simulink model "sampleModel106"  (R2022a)
settings: Solver=VariableStepAuto  StartTime=0.0  StopTime=10.0  RelTol=1e-3
undefined symbols (not defined in the file): DiscIntNeverNeededParam, magnitude, Newton, Raphson
libraries: simulink x379, slpidlib x89
(part 6 of 16)

== system sampleModel106/cfblk86/cfblk12/cfblk6 ==
  cfblk1 : Inport
  cfblk10 : Inport  Port=2
  cfblk11 : Inport  Port=3
  cfblk{14..17} (4 alike) : Delay
  cfblk3 : Delay  ShowEnablePort=on
      settings: InputPortMap=u0,e6
  cfblk4 : slpidlib/PID Controller (2DOF)  Controller=PID  Form=Parallel  TimeDomain=Discrete-time  UseExternalTs=off  SampleTime=-1  IntegratorMethod=Forward Euler  FilterMethod=Forward Euler  ControllerParametersSource=internal  P=1  I=1  UseKiTs=off  D=0  N=100  UseFilter=on  b=1  c=1  TunerSelectOption=Transfer Function Based (PID Tuner App)  InitialConditionSource=internal  InitialConditionForIntegrator=0  InitialConditionForFilter=0  DifferentiatorICPrevScaledInput=0  ExternalReset=none  TrackingMode=off  Kt=1  LimitOutput=off  SatLimitsSource=internal  UpperSaturationLimit=inf  LowerSaturationLimit=-inf  LinearizeAsGain=off  AntiWindupMode=none  Kb=1  POutMin=[]  POutMax=[]  IOutMin=[]  IOutMax=[]  DOutMin=[]  DOutMax=[]  NOutMin=[]  NOutMax=[]  bOutMin=[]  bOutMax=[]  cOutMin=[]  cOutMax=[]  SumOutMin=[]  SumOutMax=[]  SaturationOutMin=[]  SaturationOutMax=[]  PParamMin=[]  PParamMax=[]  IParamMin=[]  IParamMax=[]  DParamMin=[]  DParamMax=[]  NParamMin=[]  NParamMax=[]  bParamMin=[]  bParamMax=[]  cParamMin=[]  cParamMax=[]  KbParamMin=[]  KbParamMax=[]  KtParamMin=[]  KtParamMax=[]  KbOutMin=[]  KbOutMax=[]  KtOutMin=[]  KtOutMax=[]  IntegratorOutMin=[]  IntegratorOutMax=[]  FilterOutMin=[]  FilterOutMax=[]  SumI1OutMin=[]  SumI1OutMax=[]  SumI2OutMin=[]  SumI2OutMax=[]  SumI3OutMin=[]  SumI3OutMax=[]  SumI4OutMin=[]  SumI4OutMax=[]  SumDOutMin=[]  SumDOutMax=[]  Sum1OutMin=[]  Sum1OutMax=[]  Sum2OutMin=[]  Sum2OutMax=[]  Sum3OutMin=[]  Sum3OutMax=[]  DifferentiatorOutMin=[]  DifferentiatorOutMax=[]  FilterDiffOutCoefMin=[]  FilterDiffOutCoefMax=[]  ReciprocalOutMin=[]  ReciprocalOutMax=[]  SumDenOutMin=[]  SumDenOutMax=[]  SumNumOutMin=[]  SumNumOutMax=[]  DivideOutMin=[]  DivideOutMax=[]  UdiffTsProdOutMin=[]  UdiffTsProdOutMax=[]  NTsProdOutMin=[]  NTsProdOutMax=[]  UintegralTsProdOutMin=[]  UintegralTsProdOutMax=[]  UngainTsProdOutMin=[]  UngainTsProdOutMax=[]  IntegratorContinuousStateAttributes=''  IntegratorStateMustResolveToSignalObject=off  IntegratorRTWStateStorageClass=Auto  FilterContinuousStateAttributes=''  FilterStateMustResolveToSignalObject=off  FilterRTWStateStorageClass=Auto  ParallelPVariant=InternalParameters  IdealPVariant=Disabled  IVariant=InternalParameters  DVariant=InternalParameters  bVariant=InternalParameters  cVariant=InternalParameters  IntegratorVariant=Discrete  SatVariant=Disabled  AWVariant=Passthrough  PCopyVariant=Disabled  TRVariant=Disabled  FdbkBlocksVariant=Forward  IdealPFdbkVariant=Disabled  SatFdbkVariant=Disabled  DerivativeFilterVariant=ForwardEulerFilter  NVariant=InternalParameters  NCopyVariant=Disabled  FilterICVariant=InternalICsFilter  IntegratorICVariant=InternalICs  ExternalResetVariant=Disabled  TRSumVariant=Passthrough  SumFdbkVariant=Disabled  SumVariant=Sum_PID  TsampFilterVariant=InternalTs  TsampNgainVariant=Passthrough  TsampIntegralVariant=Passthrough  ExternalSaturationOutDataTypeStr=Inherit: Same as second input
      settings: SourceProductBaseCode=SL
  cfblk5 : Signum
  cfblk6 : Subsystem
  cfblk7 : Subsystem
  cfblk8 : Subsystem
  cfblk9 : Subsystem
  cfblk2 : Outport
  cfblk12 : Outport  Port=2
  cfblk13 : Outport  Port=3
  wires:
  cfblk10/1 -> cfblk9/1(cfblk1)
  cfblk7/1(cfblk2) -> cfblk9/2(cfblk7)
  cfblk7/2(cfblk9) -> cfblk8/1(cfblk1)
  cfblk4/1 -> cfblk3/1, cfblk7/3(cfblk8)
  cfblk8/2(cfblk8) -> cfblk2/1
  cfblk11/1 -> cfblk12/1
  cfblk3/1 -> cfblk5/1
  cfblk1/1 -> cfblk4/1
  cfblk5/1 -> cfblk9/3(cfblk8)
  cfblk7/3(cfblk10) -> cfblk9/4(cfblk9)
  cfblk9/2(cfblk10) -> cfblk6/1(cfblk1)
  cfblk6/1(cfblk2) -> cfblk13/1
  cfblk9/1(cfblk2) -> cfblk14/1
  cfblk14/1 -> cfblk3/2
  cfblk8/1(cfblk2) -> cfblk15/1
  cfblk15/1 -> cfblk7/1(cfblk1)
  cfblk8/3(cfblk9) -> cfblk16/1
  cfblk16/1 -> cfblk7/2(cfblk7)
  cfblk7/4(cfblk11) -> cfblk17/1
  cfblk17/1 -> cfblk4/2

== system sampleModel106/cfblk86/cfblk12/cfblk7 ==
  cfblk1 : Inport
  cfblk9 : Inport  Port=2
  cfblk10 : Inport  Port=3
  cfblk11 : Inport  Port=4
  cfblk12 : Inport  Port=5
  cfblk13 : Inport  Port=6
  cfblk15 : Delay
  cfblk16 : Delay
  cfblk17 : Delay
  cfblk3 : Abs  SaturateOnIntegerOverflow=off
  cfblk4 : Sum  Inputs=-+
  cfblk5 : DotProduct  OutDataTypeStr=Inherit: Inherit via internal rule
  cfblk6 : ComplexToMagnitudeAngle
  cfblk7 : Subsystem
  cfblk8 : Subsystem
  cfblk2 : Outport
  cfblk14 : Outport  Port=2
  wires:
  cfblk1/1 -> cfblk5/1
  cfblk7/1(cfblk2) -> cfblk3/1
  cfblk12/1 -> cfblk4/1
  cfblk13/1 -> cfblk4/2
  cfblk9/1 -> cfblk14/1
  cfblk11/1 -> cfblk6/1
  cfblk4/1 -> cfblk7/2(cfblk12)
  cfblk10/1 -> cfblk2/1
  cfblk5/1 -> cfblk8/2(cfblk11)
  cfblk6/1 -> cfblk7/3(cfblk13)
  cfblk8/1(cfblk2) -> cfblk7/4(cfblk14)
  cfblk3/1 -> cfblk15/1
  cfblk15/1 -> cfblk7/1(cfblk1)
  cfblk7/2(cfblk15) -> cfblk16/1
  cfblk16/1 -> cfblk5/2
  cfblk7/3(cfblk16) -> cfblk17/1
  cfblk17/1 -> cfblk8/1(cfblk1)

== system sampleModel106/cfblk86/cfblk12/cfblk8 ==
  cfblk1 : Inport
  cfblk11 : Inport  Port=2
  cfblk12 : Inport  Port=3
  cfblk10 : Subsystem
  cfblk13 : Delay
  cfblk3 : Delay
  cfblk4 : simulink/Discrete/Transfer Fcn First Order  PoleZ=0.95  ICPrevOutput=0.0  DoSatur=off
  cfblk5 : DiscreteFilter
  cfblk6 : ComplexToMagnitudeAngle
  cfblk7 : Abs  SaturateOnIntegerOverflow=off
  cfblk8 : Sqrt
  cfblk9 : Constant  Value=[-768190437.472852]  SampleTime=1
  cfblk2 : Outport
  wires:
  cfblk1/1 -> cfblk10/2(cfblk7)
  cfblk4/1 -> cfblk3/1
  cfblk11/1 -> cfblk6/1
  cfblk10/1(cfblk2) -> cfblk4/1
  cfblk10/2(cfblk11) -> cfblk2/1
  cfblk12/1 -> cfblk10/3(cfblk8)
  cfblk5/1 -> cfblk10/4(cfblk9)
  cfblk10/3(cfblk12) -> cfblk8/1
  cfblk9/1 -> cfblk7/1
  cfblk6/1 -> cfblk5/1
  cfblk7/1 -> cfblk10/5(cfblk10)
  cfblk3/1 -> cfblk13/1
  cfblk13/1 -> cfblk10/1(cfblk1)

== system sampleModel106/cfblk86/cfblk12/cfblk9 ==
  cfblk1 : Inport
  cfblk8 : Inport  Port=2
  cfblk10 : Delay
  cfblk11 : Delay
  cfblk3 : simulink/Discrete/Difference  ICPrevInput=0.0  OutMin=[]  OutMax=[]  OutDataTypeStr=Inherit: Inherit via back propagation  OutDataType=fixdt(1, 16)  OutScaling=2^-10  DoSatur=off
  cfblk4 : simulink/Math Operations/MinMax Running Resettable  Function=min  vinit=0.0
  cfblk5 : Gain  Gain=[726512921.677245]
  cfblk6 : ComplexToMagnitudeAngle
  cfblk7 : Subsystem
  cfblk9 : Delay
  cfblk2 : Outport
  wires:
  cfblk8/1 -> cfblk7/1(cfblk1)
  cfblk3/1 -> cfblk4/1
  cfblk5/1 -> cfblk7/3(cfblk15)
  cfblk7/1(cfblk2) -> cfblk4/2
  cfblk7/2(cfblk16) -> cfblk6/1
  cfblk1/1 -> cfblk2/1
  cfblk4/1 -> cfblk9/1
  cfblk9/1 -> cfblk3/1
  cfblk6/1 -> cfblk10/1
  cfblk10/1 -> cfblk5/1
  cfblk6/2 -> cfblk11/1
  cfblk11/1 -> cfblk7/2(cfblk14)

== system sampleModel106/cfblk86/cfblk13/cfblk5 ==
  cfblk1 : Inport
  cfblk13 : Inport  Port=2
  cfblk10 : Sin  TimeSource=Use external signal  SampleTime=0
  cfblk11 : Subsystem
  cfblk12 : Subsystem
  cfblk15 : Delay
  cfblk16 : Delay
  cfblk3 : Delay  ShowEnablePort=on
      settings: InputPortMap=u0,e6
  cfblk4 : DiscreteIntegrator  SampleTime=-1  ICPrevOutput=DiscIntNeverNeededParam  ICPrevScaledInput=DiscIntNeverNeededParam
  cfblk5 : Sum  Inputs=+-
  cfblk6 : Trigonometry
  cfblk7 : Trigonometry
  cfblk8 : Sum  Inputs=|++
  cfblk9 : Reshape
  cfblk2 : Outport
  cfblk14 : Outport  Port=2
  wires:
  cfblk13/1 -> cfblk8/1, cfblk11/3(cfblk10)
  cfblk8/1 -> cfblk7/1
  cfblk11/1(cfblk2) -> cfblk12/1(cfblk1)
  cfblk10/1 -> cfblk5/1
  cfblk7/1 -> cfblk6/1, cfblk5/2
  cfblk5/1 -> cfblk9/1
  cfblk9/1 -> cfblk2/1, cfblk15/1
  cfblk3/1 -> cfblk11/1(cfblk1), cfblk11/2(cfblk9)
  cfblk4/1 -> cfblk12/2(cfblk8), cfblk14/1
  cfblk12/1(cfblk2) -> cfblk10/1
  cfblk12/2(cfblk10) -> cfblk8/2
  cfblk1/1 -> cfblk3/2, cfblk4/1
  cfblk15/1 -> cfblk12/3(cfblk9)
  cfblk6/1 -> cfblk16/1
  cfblk16/1 -> cfblk3/1

== system sampleModel106/cfblk86/cfblk13/cfblk6 ==
  cfblk1 : Inport
  cfblk7 : Inport  Port=2
  cfblk8 : Inport  Port=3
  cfblk9 : Inport  Port=4
  cfblk3 : Sum  Inputs=+
  cfblk4 : Sum  Inputs=+
  cfblk5 : Constant  Value=[176043133.262875]  SampleTime=1
  cfblk6 : Subsystem
  cfblk2 : Outport
  wires:
  cfblk9/1 -> cfblk2/1
  cfblk8/1 -> cfblk3/1
  cfblk4/1 -> cfblk6/1(cfblk1)
  cfblk3/1 -> cfblk4/1
  cfblk5/1 -> cfblk6/2(cfblk5)

== system sampleModel106/cfblk86/cfblk13/cfblk7 ==
  cfblk1 : Inport
  cfblk7 : Inport  Port=2
  cfblk8 : Inport  Port=3
  cfblk10 : Delay
  cfblk3 : Constant  Value=[-929390483.160695]  SampleTime=1
  cfblk4 : Subsystem
  cfblk5 : Subsystem
  cfblk6 : Subsystem
  cfblk9 : Delay
  cfblk2 : Outport
  wires:
  cfblk8/1 -> cfblk4/1(cfblk1)
  cfblk5/1(cfblk2) -> cfblk4/2(cfblk11)
  cfblk1/1 -> cfblk2/1
  cfblk3/1 -> cfblk5/1(cfblk1)
  cfblk5/2(cfblk12) -> cfblk6/1(cfblk1)
  cfblk7/1 -> cfblk6/2(cfblk13)
  cfblk4/1(cfblk2) -> cfblk9/1
  cfblk9/1 -> cfblk5/3(cfblk11)
  cfblk6/1(cfblk2) -> cfblk10/1
  cfblk10/1 -> cfblk5/2(cfblk10)

== system sampleModel106/cfblk86/cfblk9/cfblk8 ==
  cfblk1 : Inport
  cfblk10 : Subsystem
  cfblk11 : Subsystem
  cfblk{3,12..15} (5 alike) : Delay
  cfblk4 : DiscreteStateSpace  SampleTime=-1
  cfblk5 : Product
  cfblk6 : Math  Operator=log10
  cfblk7 : ComplexToMagnitudeAngle
  cfblk8 : Subsystem
  cfblk9 : Subsystem
  cfblk2 : Outport
  wires:
  cfblk10/1(cfblk2) -> cfblk9/2(cfblk13)
  cfblk3/1 -> cfblk4/1, cfblk2/1
  cfblk6/1 -> cfblk3/1
  cfblk7/1 -> cfblk8/1(cfblk1)
  cfblk8/1(cfblk2) -> cfblk9/3(cfblk14)
  cfblk9/1(cfblk2) -> cfblk11/1(cfblk1)
  cfblk1/1 -> cfblk6/1, cfblk8/3(cfblk7), cfblk8/4(cfblk8), cfblk10/4(cfblk11)
  cfblk9/2(cfblk15) -> cfblk11/2(cfblk11)
  cfblk8/2(cfblk12) -> cfblk5/1
  cfblk7/2 -> cfblk10/1(cfblk1), cfblk10/3(cfblk10), cfblk8/7(cfblk11)
  cfblk10/3(cfblk14) -> cfblk14/1, cfblk15/1
  cfblk4/1 -> cfblk7/1, cfblk8/6(cfblk10)
  cfblk5/1 -> cfblk10/2(cfblk9), cfblk10/5(cfblk12)
  cfblk11/1(cfblk2) -> cfblk12/1
  cfblk12/1 -> cfblk9/1(cfblk1)
  cfblk10/2(cfblk13) -> cfblk13/1
  cfblk13/1 -> cfblk8/2(cfblk6)
  cfblk14/1 -> cfblk5/2
  cfblk15/1 -> cfblk8/5(cfblk9)

== system sampleModel106/cfblk87/cfblk7/cfblk10 ==
  cfblk1 : Inport
  cfblk6 : Inport  Port=2
  cfblk3 : Assignment  DiagnosticForDimensions=Warning  IndexOptions=Index vector (dialog)  Indices=1  OutputSizes=1
  cfblk4 : Constant  Value=[-447952016.572261]  SampleTime=1
  cfblk5 : Subsystem
  cfblk8 : Delay
  cfblk2 : Outport
  cfblk7 : Outport  Port=2
  wires:
  cfblk6/1 -> cfblk7/1
  cfblk4/1 -> cfblk2/1, cfblk5/3(cfblk15)
  cfblk5/1(cfblk2) -> cfblk3/1
  cfblk1/1 -> cfblk5/2(cfblk14)
  cfblk5/2(cfblk16) -> cfblk3/2
  cfblk3/1 -> cfblk8/1
  cfblk8/1 -> cfblk5/1(cfblk1)

== system sampleModel106/cfblk87/cfblk7/cfblk11 ==
  cfblk1 : Inport
  cfblk7 : Inport  Port=2
  cfblk3 : Product  Inputs=**
  cfblk4 : Reshape
  cfblk5 : Constant  Value=[-816487384.048334]  SampleTime=1
  cfblk6 : Subsystem
  cfblk2 : Outport
  cfblk8 : Outport  Port=2
  wires:
  cfblk5/1 -> cfblk4/1
  cfblk6/1(cfblk2) -> cfblk3/1
  cfblk1/1 -> cfblk2/1
  cfblk4/1 -> cfblk3/2
  cfblk7/1 -> cfblk6/1(cfblk1)
  cfblk3/1 -> cfblk8/1

== system sampleModel106/cfblk87/cfblk8/cfblk10 ==
  cfblk1 : Inport
  cfblk10 : Subsystem  TreatAsAtomicUnit=on
  cfblk11 : Subsystem  TreatAsAtomicUnit=on
  cfblk{12..18} (7 alike) : Delay
  cfblk3 : simulink/Discrete/Tapped Delay  vinit=0.0  samptime=-1  NumDelays=1  DelayOrder=Oldest  includeCurrent=off
  cfblk4 : Subsystem
  cfblk5 : Subsystem
  cfblk6 : If  IfExpression=u1 >= 0  SampleTime=1
  cfblk7 : If  IfExpression=u1 >= 0  SampleTime=1
  cfblk8 : Subsystem  TreatAsAtomicUnit=on
  cfblk9 : Subsystem  TreatAsAtomicUnit=on
  cfblk2 : Outport
  wires:
  cfblk11/1(cfblk2) -> cfblk4/1(cfblk1)
  cfblk10/1(cfblk2) -> cfblk5/1(cfblk1), cfblk18/1
  cfblk1/1 -> cfblk6/1, cfblk11/2(cfblk10), cfblk2/1
  cfblk9/1(cfblk2) -> cfblk3/1
  cfblk5/2(cfblk15) -> cfblk16/1, cfblk17/1
  cfblk8/1(cfblk2) -> cfblk11/1(cfblk1)
  cfblk6/1 -> cfblk8/Action
  cfblk6/2 -> cfblk9/Action
  cfblk7/1 -> cfblk10/Action
  cfblk7/2 -> cfblk11/Action
  cfblk4/1(cfblk2) -> cfblk12/1
  cfblk12/1 -> cfblk10/1(cfblk1)
  cfblk5/1(cfblk2) -> cfblk13/1
  cfblk13/1 -> cfblk9/2(cfblk14)
  cfblk3/1 -> cfblk14/1
  cfblk14/1 -> cfblk9/1(cfblk1)
  cfblk9/2(cfblk15) -> cfblk15/1
  cfblk15/1 -> cfblk7/1
  cfblk16/1 -> cfblk8/1(cfblk1)
  cfblk17/1 -> cfblk11/3(cfblk11)
  cfblk18/1 -> cfblk8/2(cfblk9)

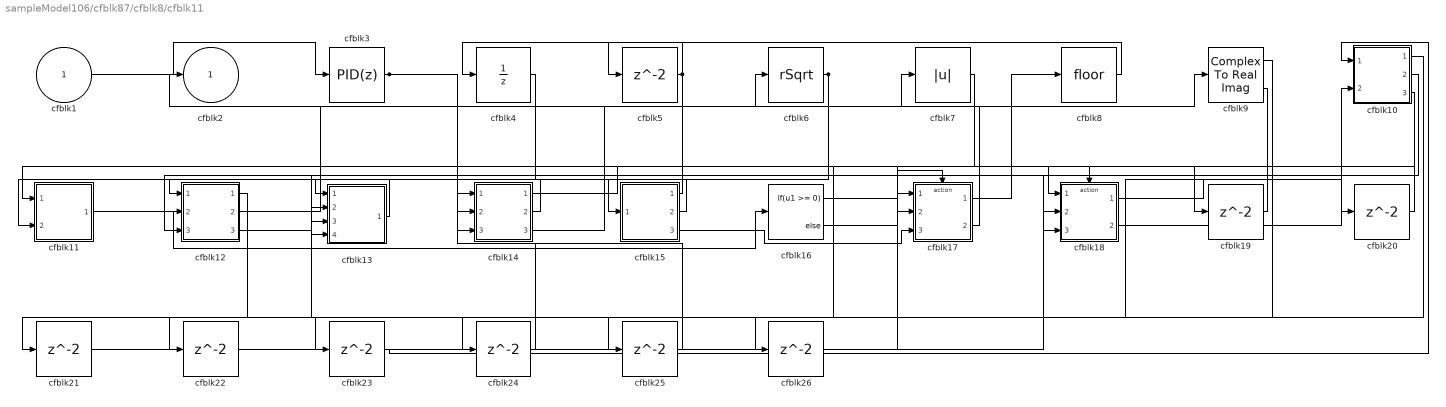
== system sampleModel106/cfblk87/cfblk8/cfblk11 ==
  cfblk1 : Inport
  cfblk10 : Subsystem
  cfblk11 : Subsystem
  cfblk12 : Subsystem
  cfblk13 : Subsystem
  cfblk14 : Subsystem
  cfblk15 : Subsystem
  cfblk16 : If  IfExpression=u1 >= 0  SampleTime=1
  cfblk17 : Subsystem  TreatAsAtomicUnit=on
  cfblk18 : Subsystem  TreatAsAtomicUnit=on
  cfblk{5,19..26} (9 alike) : Delay
  cfblk3 : slpidlib/PID Controller  Controller=PID  Form=Parallel  TimeDomain=Discrete-time  UseExternalTs=off  SampleTime=-1  IntegratorMethod=Forward Euler  FilterMethod=Forward Euler  ControllerParametersSource=internal  P=1  I=1  UseKiTs=off  D=0  N=100  UseFilter=on  TunerSelectOption=Transfer Function Based (PID Tuner App)  InitialConditionSource=internal  InitialConditionForIntegrator=0  InitialConditionForFilter=0  DifferentiatorICPrevScaledInput=0  ExternalReset=none  TrackingMode=off  Kt=1  LimitOutput=off  SatLimitsSource=internal  UpperSaturationLimit=inf  LowerSaturationLimit=-inf  LinearizeAsGain=off  AntiWindupMode=none  Kb=1  POutMin=[]  POutMax=[]  IOutMin=[]  IOutMax=[]  DOutMin=[]  DOutMax=[]  NOutMin=[]  NOutMax=[]  SumOutMin=[]  SumOutMax=[]  SaturationOutMin=[]  SaturationOutMax=[]  PParamMin=[]  PParamMax=[]  IParamMin=[]  IParamMax=[]  DParamMin=[]  DParamMax=[]  NParamMin=[]  NParamMax=[]  KbParamMin=[]  KbParamMax=[]  KtParamMin=[]  KtParamMax=[]  KbOutMin=[]  KbOutMax=[]  KtOutMin=[]  KtOutMax=[]  IntegratorOutMin=[]  IntegratorOutMax=[]  FilterOutMin=[]  FilterOutMax=[]  SumI1OutMin=[]  SumI1OutMax=[]  SumI2OutMin=[]  SumI2OutMax=[]  SumI3OutMin=[]  SumI3OutMax=[]  SumI4OutMin=[]  SumI4OutMax=[]  SumDOutMin=[]  SumDOutMax=[]  DifferentiatorOutMin=[]  DifferentiatorOutMax=[]  FilterDiffOutCoefMin=[]  FilterDiffOutCoefMax=[]  ReciprocalOutMin=[]  ReciprocalOutMax=[]  SumDenOutMin=[]  SumDenOutMax=[]  SumNumOutMin=[]  SumNumOutMax=[]  DivideOutMin=[]  DivideOutMax=[]  UdiffTsProdOutMin=[]  UdiffTsProdOutMax=[]  NTsProdOutMin=[]  NTsProdOutMax=[]  UintegralTsProdOutMin=[]  UintegralTsProdOutMax=[]  UngainTsProdOutMin=[]  UngainTsProdOutMax=[]  IntegratorContinuousStateAttributes=''  IntegratorStateMustResolveToSignalObject=off  IntegratorRTWStateStorageClass=Auto  FilterContinuousStateAttributes=''  FilterStateMustResolveToSignalObject=off  FilterRTWStateStorageClass=Auto  ParallelPVariant=InternalParameters  IdealPVariant=Disabled  IVariant=InternalParameters  DVariant=InternalParameters  IntegratorVariant=Discrete  SatVariant=Disabled  AWVariant=Passthrough  PCopyVariant=Disabled  TRVariant=Disabled  FdbkBlocksVariant=Forward  IdealPFdbkVariant=Disabled  SatFdbkVariant=Disabled  DerivativeFilterVariant=ForwardEulerFilter  NVariant=InternalParameters  NCopyVariant=Disabled  FilterICVariant=InternalICsFilter  IntegratorICVariant=InternalICs  ExternalResetVariant=Disabled  TRSumVariant=Passthrough  SumFdbkVariant=Disabled  SumVariant=Sum_PID  TsampFilterVariant=InternalTs  TsampNgainVariant=Passthrough  TsampIntegralVariant=Passthrough  ExternalSaturationOutDataTypeStr=Inherit: Same as second input  aMode=0
  cfblk4 : UnitDelay  SampleTime=-1  HasFrameUpgradeWarning=on
  cfblk6 : Sqrt  Operator=rSqrt  AlgorithmType=Newton-Raphson
  cfblk7 : Abs  SaturateOnIntegerOverflow=off
  cfblk8 : Rounding
  cfblk9 : ComplexToRealImag
  cfblk2 : Outport
  wires:
  cfblk5/1 -> cfblk4/1, cfblk13/3(cfblk10)
  cfblk1/1 -> cfblk3/1
  cfblk11/1(cfblk2) -> cfblk16/1
  cfblk17/1(cfblk2) -> cfblk8/1
  cfblk6/1 -> cfblk2/1, cfblk13/4(cfblk11)
  cfblk12/2(cfblk13) -> cfblk9/1
  cfblk17/2(cfblk13) -> cfblk6/1
  cfblk15/1(cfblk2) -> cfblk11/2(cfblk7)
  cfblk3/1 -> cfblk15/1(cfblk1), cfblk18/3(cfblk8)
  cfblk13/1(cfblk2) -> cfblk12/1(cfblk1)
  cfblk18/2(cfblk9) -> cfblk10/2(cfblk13)
  cfblk4/1 -> cfblk14/3(cfblk11)
  cfblk15/2(cfblk10) -> cfblk13/1(cfblk1)
  cfblk8/1 -> cfblk5/1
  cfblk14/2(cfblk12) -> cfblk12/2(cfblk11)
  cfblk14/3(cfblk13) -> cfblk7/1
  cfblk15/3(cfblk11) -> cfblk17/3(cfblk12)
  cfblk10/2(cfblk14) -> cfblk12/3(cfblk12)
  cfblk10/3(cfblk15) -> cfblk13/2(cfblk9)
  cfblk16/1 -> cfblk17/Action
  cfblk16/2 -> cfblk18/Action
  cfblk14/1(cfblk2) -> cfblk19/1
  cfblk19/1 -> cfblk18/1(cfblk1)
  cfblk18/1(cfblk2) -> cfblk20/1
  cfblk20/1 -> cfblk11/1(cfblk1)
  cfblk10/1(cfblk2) -> cfblk21/1
  cfblk21/1 -> cfblk18/2(cfblk7)
  cfblk12/1(cfblk2) -> cfblk22/1
  cfblk22/1 -> cfblk17/1(cfblk1)
  cfblk9/1 -> cfblk23/1
  cfblk23/1 -> cfblk10/1(cfblk1)
  cfblk9/2 -> cfblk24/1
  cfblk24/1 -> cfblk14/2(cfblk10)
  cfblk12/3(cfblk14) -> cfblk25/1
  cfblk25/1 -> cfblk14/1(cfblk1)
  cfblk7/1 -> cfblk26/1
  cfblk26/1 -> cfblk17/2(cfblk11)

== system sampleModel106/cfblk87/cfblk9/cfblk13 ==
  cfblk1 : Inport
  cfblk10 : Subsystem  TreatAsAtomicUnit=on
  cfblk11 : Delay
  cfblk12 : Delay
  cfblk13 : Delay
  cfblk3 : DiscreteFir
  cfblk4 : UnitDelay  SampleTime=-1  HasFrameUpgradeWarning=on
  cfblk5 : Delay  DelayLengthSource=Input port
      settings: InputPortMap=u0,p1
  cfblk6 : Sum  Inputs=+-
  cfblk7 : If  IfExpression=u1 >= 0  SampleTime=1
  cfblk9 : Subsystem  TreatAsAtomicUnit=on
  cfblk2 : Outport
  cfblk8 : Outport  Port=2
  wires:
  cfblk1/1 -> cfblk9/1(cfblk1), cfblk4/1
  cfblk10/1(cfblk2) -> cfblk8/1
  cfblk4/1 -> cfblk10/1(cfblk1), cfblk10/3(cfblk12)
  cfblk9/1(cfblk2) -> cfblk6/1, cfblk5/2, cfblk10/2(cfblk11)
  cfblk5/1 -> cfblk3/1, cfblk2/1
  cfblk3/1 -> cfblk6/2, cfblk12/1, cfblk13/1
  cfblk7/1 -> cfblk9/Action
  cfblk7/2 -> cfblk10/Action
  cfblk6/1 -> cfblk11/1
  cfblk11/1 -> cfblk9/2(cfblk8)
  cfblk12/1 -> cfblk7/1
  cfblk13/1 -> cfblk5/1

== system sampleModel106/cfblk87/cfblk9/cfblk14 ==
  cfblk1 : Inport
  cfblk8 : Inport  Port=2
  cfblk3 : DiscreteFir
  cfblk4 : simulink/Math Operations/Slider Gain  gain=1  low=0  high=2
  cfblk5 : Subsystem
  cfblk6 : Subsystem
  cfblk7 : Subsystem
  cfblk9 : Delay
  cfblk2 : Outport
  wires:
  cfblk5/1(cfblk2) -> cfblk3/1
  cfblk8/1 -> cfblk6/2(cfblk10)
  cfblk7/2(cfblk9) -> cfblk4/1
  cfblk3/1 -> cfblk7/1(cfblk1)
  cfblk1/1 -> cfblk6/3(cfblk11)
  cfblk4/1 -> cfblk2/1
  cfblk6/1(cfblk2) -> cfblk5/1(cfblk1)
  cfblk6/2(cfblk12) -> cfblk7/2(cfblk8)
  cfblk7/1(cfblk2) -> cfblk9/1
  cfblk9/1 -> cfblk6/1(cfblk1)

== system sampleModel106/cfblk87/cfblk9/cfblk15 ==
  cfblk1 : Inport
  cfblk16 : Inport  Port=2
  cfblk17 : Inport  Port=3
  cfblk10 : Constant  Value=[53505652.263699]  SampleTime=1
  cfblk11 : Subsystem
  cfblk12 : Subsystem
  cfblk13 : Subsystem
  cfblk14 : Subsystem
  cfblk15 : If  IfExpression=u1 >= 0  SampleTime=1
  cfblk18 : Subsystem  TreatAsAtomicUnit=on
  cfblk19 : Subsystem  TreatAsAtomicUnit=on
  cfblk{4,20..23} (5 alike) : Delay
  cfblk3 : DiscreteStateSpace  SampleTime=-1
  cfblk5 : ComplexToMagnitudeAngle
  cfblk6 : Sqrt
  cfblk7 : Sum  Inputs=+
  cfblk8 : simulink/Math Operations/MinMax Running Resettable  Function=min  vinit=0.0
  cfblk9 : Constant  Value=[-649991025.469007]  SampleTime=1
  cfblk2 : Outport
  wires:
  cfblk7/1 -> cfblk19/1(cfblk1)
  cfblk13/1(cfblk2) -> cfblk12/1(cfblk1)
  cfblk3/1 -> cfblk19/2(cfblk9)
  cfblk19/1(cfblk2) -> cfblk6/1
  cfblk10/1 -> cfblk7/1
  cfblk11/1(cfblk2) -> cfblk4/1
  cfblk19/2(cfblk10) -> cfblk2/1
  cfblk16/1 -> cfblk11/1(cfblk1)
  cfblk1/1 -> cfblk11/2(cfblk13)
  cfblk4/1 -> cfblk8/1
  cfblk12/2(cfblk10) -> cfblk14/1(cfblk1)
  cfblk19/3(cfblk11) -> cfblk18/1(cfblk1)
  cfblk17/1 -> cfblk8/2
  cfblk18/1(cfblk2) -> cfblk5/1
  cfblk8/1 -> cfblk3/1
  cfblk5/2 -> cfblk13/1(cfblk1)
  cfblk18/2(cfblk12) -> cfblk14/2(cfblk12)
  cfblk12/4(cfblk12) -> cfblk14/3(cfblk13)
  cfblk15/1 -> cfblk18/Action
  cfblk15/2 -> cfblk19/Action
  cfblk5/1 -> cfblk20/1
  cfblk20/1 -> cfblk18/2(cfblk11)
  cfblk12/1(cfblk2) -> cfblk21/1
  cfblk21/1 -> cfblk15/1
  cfblk14/1(cfblk2) -> cfblk22/1
  cfblk22/1 -> cfblk12/2(cfblk9)
  cfblk12/3(cfblk11) -> cfblk23/1
  cfblk23/1 -> cfblk13/2(cfblk8)

== system sampleModel106/cfblk74/cfblk10/cfblk11/cfblk10 ==
  cfblk1 : Inport
  cfblk12 : Inport  Port=2
  cfblk13 : Inport  Port=3
  cfblk10 : Constant  Value=[-540089913.377910]  SampleTime=1
  cfblk11 : Constant  Value=[-943634033.033657]  SampleTime=1
  cfblk15 : Delay  SampleTime=1
  cfblk3 : DiscreteFilter  SampleTime=1
  cfblk4 : UnitDelay  HasFrameUpgradeWarning=on
  cfblk5 : Polyval  Coefs=[ +2.081618890e-019, -1.441693666e-014, +4.719686976e-010, -8.536869453e-006, +1.621573104e-001, -8.087801117e+001 ]
  cfblk6 : Signum
  cfblk7 : Sum  Inputs=+-
  cfblk8 : DotProduct  OutDataTypeStr=Inherit: Inherit via internal rule
  cfblk9 : Signum
  cfblk2 : Outport
  cfblk14 : Outport  Port=2
  wires:
  cfblk5/1 -> cfblk4/1
  cfblk7/1 -> cfblk9/1
  cfblk1/1 -> cfblk7/1
  cfblk13/1 -> cfblk3/1
  cfblk11/1 -> cfblk6/1
  cfblk3/1 -> cfblk14/1
  cfblk9/1 -> cfblk5/1
  cfblk12/1 -> cfblk2/1
  cfblk6/1 -> cfblk8/1
  cfblk10/1 -> cfblk8/2
  cfblk4/1 -> cfblk15/1
  cfblk15/1 -> cfblk7/2

== system sampleModel106/cfblk74/cfblk10/cfblk11/cfblk16 ==
  cfblk1 : Inport
  cfblk11 : Inport  Port=2
  Action Port : ActionPort  ActionPortLabel=if(u1 >= 0)
  cfblk10 : Constant  Value=[-263193353.112498]  SampleTime=1
  cfblk14 : Delay
  cfblk3 : DiscreteStateSpace  SampleTime=-1
  cfblk4 : Rounding
  cfblk5 : simulink/Math Operations/Slider Gain  gain=1  low=0  high=2
  cfblk6 : Sin  TimeSource=Use external signal  SampleTime=0
  cfblk7 : simulink/Math Operations/Slider Gain  gain=1  low=0  high=2
  cfblk8 : Sum  Inputs=+-
  cfblk9 : Constant  Value=[659902283.090515]  SampleTime=1
  cfblk2 : Outport
  cfblk12 : Outport  Port=2
  cfblk13 : Outport  Port=3
  wires:
  cfblk3/1 -> cfblk5/1
  cfblk11/1 -> cfblk2/1
  cfblk4/1 -> cfblk8/1
  cfblk1/1 -> cfblk13/1
  cfblk5/1 -> cfblk12/1
  cfblk9/1 -> cfblk4/1
  cfblk10/1 -> cfblk7/1
  cfblk7/1 -> cfblk3/1
  cfblk8/1 -> cfblk6/1
  cfblk6/1 -> cfblk14/1
  cfblk14/1 -> cfblk8/2

== system sampleModel106/cfblk74/cfblk10/cfblk11/cfblk17 ==
  cfblk1 : Inport
  cfblk13 : Inport  Port=2
  cfblk14 : Inport  Port=3
  cfblk15 : Inport  Port=4
  cfblk16 : Inport  Port=5
  Action Port : ActionPort  ActionPortLabel=else
  cfblk10 : Sum  Inputs=-+
  cfblk11 : Constant  Value=[515772404.945346]  SampleTime=1
  cfblk12 : Constant  Value=[215448082.062635]  SampleTime=1
  cfblk17 : Delay
  cfblk3 : UnitDelay  SampleTime=-1  HasFrameUpgradeWarning=on
  cfblk4 : simulink/Discrete/Transfer Fcn First Order  PoleZ=0.95  ICPrevOutput=0.0  DoSatur=off
  cfblk5 : Sqrt  Operator=rSqrt  AlgorithmType=Newton-Raphson
  cfblk6 : Bias  Bias=[206614008.129660]  SaturateOnIntegerOverflow=off
  cfblk7 : Polyval  Coefs=[ +2.081618890e-019, -1.441693666e-014, +4.719686976e-010, -8.536869453e-006, +1.621573104e-001, -8.087801117e+001 ]
  cfblk8 : Sum  Inputs=--
  cfblk9 : PermuteDimensions
  cfblk2 : Outport
  wires:
  cfblk4/1 -> cfblk6/1
  cfblk7/1 -> cfblk9/1
  cfblk13/1 -> cfblk4/1
  cfblk3/1 -> cfblk2/1
  cfblk9/1 -> cfblk10/1
  cfblk16/1 -> cfblk3/1
  cfblk5/1 -> cfblk8/1
  cfblk6/1 -> cfblk5/1
  cfblk11/1 -> cfblk10/2
  cfblk12/1 -> cfblk8/2
  cfblk10/1 -> cfblk17/1
  cfblk17/1 -> cfblk7/1

== system sampleModel106/cfblk74/cfblk10/cfblk11/cfblk18 ==
  cfblk1 : Inport
  cfblk12 : Inport  Port=2
  cfblk13 : Inport  Port=3
  cfblk14 : Inport  Port=4
  cfblk15 : Inport  Port=5
  Action Port : ActionPort  ActionPortLabel=if(u1 >= 0)
  cfblk10 : ComplexToRealImag
  cfblk11 : Trigonometry
  cfblk3 : DiscreteFilter
  cfblk4 : simulink/Discrete/Transfer Fcn First Order  PoleZ=0.95  ICPrevOutput=0.0  DoSatur=off
  cfblk5 : Delay  ShowEnablePort=on
      settings: InputPortMap=u0,e6
  cfblk6 : simulink/Discrete/Difference  ICPrevInput=0.0  OutMin=[]  OutMax=[]  OutDataTypeStr=Inherit: Inherit via back propagation  OutDataType=fixdt(1, 16)  OutScaling=2^-10  DoSatur=off
  cfblk7 : ComplexToMagnitudeAngle
  cfblk8 : MinMax  Function=max
  cfblk9 : Rounding
  cfblk2 : Outport
  cfblk16 : Outport  Port=2
  cfblk17 : Outport  Port=3
  wires:
  cfblk3/1 -> cfblk4/1
  cfblk9/1 -> cfblk8/1
  cfblk8/1 -> cfblk7/1
  cfblk11/1 -> cfblk2/1
  cfblk12/1 -> cfblk3/1
  cfblk14/1 -> cfblk11/1
  cfblk10/1 -> cfblk16/1
  cfblk4/1 -> cfblk10/1
  cfblk7/1 -> cfblk5/1
  cfblk5/1 -> cfblk17/1
  cfblk7/2 -> cfblk6/1
  cfblk10/2 -> cfblk5/2
  cfblk13/1 -> cfblk9/1

== system sampleModel106/cfblk74/cfblk10/cfblk11/cfblk19 ==
  cfblk1 : Inport
  cfblk7 : Inport  Port=2
  Action Port : ActionPort  ActionPortLabel=else
  cfblk3 : Trigonometry
  cfblk4 : Squeeze
  cfblk5 : Assignment  DiagnosticForDimensions=Warning  IndexOptions=Index vector (dialog)  Indices=1  OutputSizes=1
  cfblk6 : Sum  Inputs=-+
  cfblk8 : Delay
  cfblk2 : Outport
  wires:
  cfblk4/1 -> cfblk3/1
  cfblk7/1 -> cfblk2/1
  cfblk5/1 -> cfblk4/1
  cfblk6/1 -> cfblk5/1
  cfblk1/1 -> cfblk6/2, cfblk5/2
  cfblk3/1 -> cfblk8/1
  cfblk8/1 -> cfblk6/1

== system sampleModel106/cfblk74/cfblk10/cfblk11/cfblk9 ==
  cfblk1 : Inport
  cfblk8 : Inport  Port=2
  cfblk9 : Inport  Port=3
  cfblk3 : Delay  DelayLengthSource=Input port  SampleTime=1
      settings: InputPortMap=u0,p1
  cfblk4 : Bias  Bias=[-444008973.315964]  SaturateOnIntegerOverflow=off
  cfblk5 : UnaryMinus
  cfblk6 : Constant  Value=[658809830.773838]  SampleTime=1
  cfblk7 : Constant  Value=[994529317.523357]  SampleTime=1
  cfblk2 : Outport
  cfblk10 : Outport  Port=2
  cfblk11 : Outport  Port=3
  wires:
  cfblk6/1 -> cfblk2/1
  cfblk9/1 -> cfblk5/1
  cfblk8/1 -> cfblk10/1
  cfblk4/1 -> cfblk11/1
  cfblk5/1 -> cfblk3/1
  cfblk1/1 -> cfblk3/2
  cfblk7/1 -> cfblk4/1

== system sampleModel106/cfblk74/cfblk11/cfblk6/cfblk10 ==
  cfblk1 : Inport
  cfblk12 : Inport  Port=2
  cfblk13 : Inport  Port=3
  cfblk14 : Inport  Port=4
  cfblk15 : Inport  Port=5
  cfblk10 : Constant  Value=[-7215338.026808]  SampleTime=1
  cfblk11 : Constant  Value=[290313939.831306]  SampleTime=1
  cfblk3 : Delay  DelayLengthSource=Input port  SampleTime=1
      settings: InputPortMap=u0,p1
  cfblk4 : DiscreteFir  SampleTime=1
  cfblk5 : DiscreteFilter  SampleTime=1
  cfblk6 : Sqrt
  cfblk7 : Assignment  DiagnosticForDimensions=Warning  IndexOptions=Index vector (dialog)  Indices=1  OutputSizes=1
  cfblk8 : Constant  Value=[-383804505.867733]  SampleTime=1
  cfblk9 : Constant  Value=[905638390.574279]  SampleTime=1
  cfblk2 : Outport
  cfblk16 : Outport  Port=2
  cfblk17 : Outport  Port=3
  wires:
  cfblk5/1 -> cfblk17/1
  cfblk4/1 -> cfblk3/1
  cfblk13/1 -> cfblk3/2
  cfblk10/1 -> cfblk16/1
  cfblk12/1 -> cfblk6/1
  cfblk3/1 -> cfblk5/1
  cfblk15/1 -> cfblk2/1
  cfblk11/1 -> cfblk4/1
  cfblk9/1 -> cfblk7/1
  cfblk6/1 -> cfblk7/2

== system sampleModel106/cfblk74/cfblk11/cfblk6/cfblk17 ==
  cfblk1 : Inport
  cfblk13 : Inport  Port=2
  cfblk14 : Inport  Port=3
  Action Port : ActionPort  ActionPortLabel=if(u1 >= 0)
  cfblk10 : Sum  Inputs=--
  cfblk11 : ComplexToMagnitudeAngle
  cfblk12 : UnaryMinus
  cfblk16 : Delay
  cfblk3 : simulink/Discrete/Transfer Fcn Real Zero  ZeroZ=0.75  ICPrevInput=0.0  DoSatur=off
      settings: SourceProductBaseCode=SL
  cfblk4 : simulink/Discrete/Transfer Fcn Lead or Lag  PoleZ=0.95  ZeroZ=0.75  ICPrevOutput=0.0  ICPrevInput=0.0  DoSatur=off
      settings: SourceProductBaseCode=SL
  cfblk5 : Polyval  Coefs=[ +2.081618890e-019, -1.441693666e-014, +4.719686976e-010, -8.536869453e-006, +1.621573104e-001, -8.087801117e+001 ]
  cfblk6 : UnaryMinus
  cfblk7 : PermuteDimensions
  cfblk8 : Sqrt  Operator=rSqrt  AlgorithmType=Newton-Raphson
  cfblk9 : Signum
  cfblk2 : Outport
  cfblk15 : Outport  Port=2
  wires:
  cfblk8/1 -> cfblk2/1
  cfblk11/1 -> cfblk4/1
  cfblk7/1 -> cfblk6/1
  cfblk13/1 -> cfblk11/1
  cfblk6/1 -> cfblk12/1
  cfblk9/1 -> cfblk10/1
  cfblk14/1 -> cfblk5/1
  cfblk5/1 -> cfblk10/2
  cfblk3/1 -> cfblk7/1
  cfblk11/2 -> cfblk8/1
  cfblk4/1 -> cfblk9/1
  cfblk1/1 -> cfblk15/1
  cfblk12/1 -> cfblk16/1
  cfblk16/1 -> cfblk3/1

== system sampleModel106/cfblk74/cfblk11/cfblk6/cfblk18 ==
  cfblk1 : Inport
  Action Port : ActionPort  ActionPortLabel=else
  cfblk3 : Delay  ShowEnablePort=on
      settings: InputPortMap=u0,e6
  cfblk4 : Squeeze
  cfblk5 : Product  Inputs=**
  cfblk6 : Reshape
  cfblk7 : Bias  Bias=[-430206245.269602]  SaturateOnIntegerOverflow=off
  cfblk8 : Constant  Value=[-6900892.655831]  SampleTime=1
  cfblk2 : Outport
  cfblk9 : Outport  Port=2
  wires:
  cfblk6/1 -> cfblk4/1, cfblk5/1, cfblk5/2
  cfblk7/1 -> cfblk6/1
  cfblk8/1 -> cfblk3/1
  cfblk3/1 -> cfblk9/1
  cfblk4/1 -> cfblk2/1
  cfblk5/1 -> cfblk3/2
  cfblk1/1 -> cfblk7/1

== system sampleModel106/cfblk74/cfblk11/cfblk6/cfblk6 ==
  cfblk1 : Inport
  cfblk13 : Inport  Port=2
  cfblk14 : Inport  Port=3
  cfblk10 : Sqrt
  cfblk11 : Abs  SaturateOnIntegerOverflow=off
  cfblk12 : Constant  Value=[184706769.437218]  SampleTime=1
  cfblk3 : simulink/Discrete/Transfer Fcn Real Zero  ZeroZ=0.75  ICPrevInput=0.0  DoSatur=off
      settings: SourceProductBaseCode=SL
  cfblk4 : DiscreteFir  SampleTime=1
  cfblk5 : simulink/Discrete/Transfer Fcn Real Zero  ZeroZ=0.75  ICPrevInput=0.0  DoSatur=off
      settings: SourceProductBaseCode=SL
  cfblk6 : MinMax  Function=max
  cfblk7 : Sum  Inputs=--
  cfblk8 : Abs  SaturateOnIntegerOverflow=off
  cfblk9 : Polyval  Coefs=[ +2.081618890e-019, -1.441693666e-014, +4.719686976e-010, -8.536869453e-006, +1.621573104e-001, -8.087801117e+001 ]
  cfblk2 : Outport
  cfblk15 : Outport  Port=2
  cfblk16 : Outport  Port=3
  cfblk17 : Outport  Port=4
  wires:
  cfblk3/1 -> cfblk15/1
  cfblk12/1 -> cfblk11/1
  cfblk1/1 -> cfblk10/1
  cfblk9/1 -> cfblk2/1
  cfblk11/1 -> cfblk3/1
  cfblk4/1 -> cfblk9/1
  cfblk13/1 -> cfblk6/1, cfblk7/2
  cfblk6/1 -> cfblk4/1
  cfblk8/1 -> cfblk16/1
  cfblk5/1 -> cfblk17/1
  cfblk10/1 -> cfblk5/1
  cfblk14/1 -> cfblk7/1
  cfblk7/1 -> cfblk8/1

== system sampleModel106/cfblk74/cfblk11/cfblk6/cfblk7 ==
  cfblk1 : Inport
  cfblk10 : Inport  Port=2
  cfblk3 : Rounding
  cfblk4 : Rounding
  cfblk5 : Squeeze
  cfblk6 : ComplexToMagnitudeAngle
  cfblk7 : Product  Inputs=**
  cfblk8 : Sum  Inputs=--
  cfblk9 : ComplexToMagnitudeAngle
  cfblk2 : Outport
  cfblk11 : Outport  Port=2
  wires:
  cfblk8/1 -> cfblk2/1
  cfblk1/1 -> cfblk8/1
  cfblk10/1 -> cfblk3/1
  cfblk4/1 -> cfblk5/1
  cfblk9/1 -> cfblk7/1
  cfblk6/1 -> cfblk8/2
  cfblk7/1 -> cfblk11/1
  cfblk3/1 -> cfblk4/1
  cfblk6/2 -> cfblk7/2
  cfblk9/2 -> cfblk6/1
  cfblk5/1 -> cfblk9/1

== system sampleModel106/cfblk74/cfblk11/cfblk6/cfblk8 ==
  cfblk1 : Inport
  cfblk6 : Inport  Port=2
  cfblk3 : PermuteDimensions
  cfblk4 : Constant  Value=[-769911818.679232]  SampleTime=1
  cfblk5 : Constant  Value=[257449604.661901]  SampleTime=1
  cfblk2 : Outport
  cfblk7 : Outport  Port=2
  wires:
  cfblk3/1 -> cfblk2/1
  cfblk5/1 -> cfblk7/1
  cfblk6/1 -> cfblk3/1

== system sampleModel106/cfblk74/cfblk11/cfblk6/cfblk9 ==
  cfblk1 : Inport
  cfblk13 : Delay  SampleTime=1
  cfblk14 : Delay  SampleTime=1
  cfblk3 : Delay  ShowEnablePort=on  SampleTime=1
      settings: InputPortMap=u0,e6
  cfblk4 : Polyval  Coefs=[ +2.081618890e-019, -1.441693666e-014, +4.719686976e-010, -8.536869453e-006, +1.621573104e-001, -8.087801117e+001 ]
  cfblk5 : Gain  Gain=[-627357319.587642]
  cfblk6 : Rounding
  cfblk7 : ComplexToMagnitudeAngle
  cfblk8 : Math
  cfblk9 : Constant  Value=[750292379.008376]  SampleTime=1
  cfblk2 : Outport
  cfblk10 : Outport  Port=2
  cfblk11 : Outport  Port=3
  cfblk12 : Outport  Port=4
  wires:
  cfblk4/1 -> cfblk8/1
  cfblk7/1 -> cfblk6/1
  cfblk9/1 -> cfblk11/1
  cfblk8/1 -> cfblk2/1
  cfblk6/1 -> cfblk10/1, cfblk13/1
  cfblk3/1 -> cfblk4/1, cfblk5/1
  cfblk1/1 -> cfblk12/1
  cfblk5/1 -> cfblk7/1
  cfblk13/1 -> cfblk3/2
  cfblk7/2 -> cfblk14/1
  cfblk14/1 -> cfblk3/1

== system sampleModel106/cfblk74/cfblk12/cfblk6/cfblk13 ==
  cfblk1 : Inport
  cfblk10 : Inport  Port=2
  cfblk11 : Inport  Port=3
  cfblk12 : Inport  Port=4
  cfblk14 : Delay  SampleTime=1
  cfblk3 : slpidlib/PID Controller  Controller=PID  Form=Parallel  TimeDomain=Discrete-time  UseExternalTs=off  SampleTime=1  IntegratorMethod=Forward Euler  FilterMethod=Forward Euler  ControllerParametersSource=internal  P=1  I=1  UseKiTs=off  D=0  N=100  UseFilter=on  TunerSelectOption=Transfer Function Based (PID Tuner App)  InitialConditionSource=internal  InitialConditionForIntegrator=0  InitialConditionForFilter=0  DifferentiatorICPrevScaledInput=0  ExternalReset=none  TrackingMode=off  Kt=1  LimitOutput=off  SatLimitsSource=internal  UpperSaturationLimit=inf  LowerSaturationLimit=-inf  LinearizeAsGain=off  AntiWindupMode=none  Kb=1  POutMin=[]  POutMax=[]  IOutMin=[]  IOutMax=[]  DOutMin=[]  DOutMax=[]  NOutMin=[]  NOutMax=[]  SumOutMin=[]  SumOutMax=[]  SaturationOutMin=[]  SaturationOutMax=[]  PParamMin=[]  PParamMax=[]  IParamMin=[]  IParamMax=[]  DParamMin=[]  DParamMax=[]  NParamMin=[]  NParamMax=[]  KbParamMin=[]  KbParamMax=[]  KtParamMin=[]  KtParamMax=[]  KbOutMin=[]  KbOutMax=[]  KtOutMin=[]  KtOutMax=[]  IntegratorOutMin=[]  IntegratorOutMax=[]  FilterOutMin=[]  FilterOutMax=[]  SumI1OutMin=[]  SumI1OutMax=[]  SumI2OutMin=[]  SumI2OutMax=[]  SumI3OutMin=[]  SumI3OutMax=[]  SumI4OutMin=[]  SumI4OutMax=[]  SumDOutMin=[]  SumDOutMax=[]  DifferentiatorOutMin=[]  DifferentiatorOutMax=[]  FilterDiffOutCoefMin=[]  FilterDiffOutCoefMax=[]  ReciprocalOutMin=[]  ReciprocalOutMax=[]  SumDenOutMin=[]  SumDenOutMax=[]  SumNumOutMin=[]  SumNumOutMax=[]  DivideOutMin=[]  DivideOutMax=[]  UdiffTsProdOutMin=[]  UdiffTsProdOutMax=[]  NTsProdOutMin=[]  NTsProdOutMax=[]  UintegralTsProdOutMin=[]  UintegralTsProdOutMax=[]  UngainTsProdOutMin=[]  UngainTsProdOutMax=[]  IntegratorContinuousStateAttributes=''  IntegratorStateMustResolveToSignalObject=off  IntegratorRTWStateStorageClass=Auto  FilterContinuousStateAttributes=''  FilterStateMustResolveToSignalObject=off  FilterRTWStateStorageClass=Auto  ParallelPVariant=InternalParameters  IdealPVariant=Disabled  IVariant=InternalParameters  DVariant=InternalParameters  IntegratorVariant=Discrete  SatVariant=Disabled  AWVariant=Passthrough  PCopyVariant=Disabled  TRVariant=Disabled  FdbkBlocksVariant=Forward  IdealPFdbkVariant=Disabled  SatFdbkVariant=Disabled  DerivativeFilterVariant=ForwardEulerFilter  NVariant=InternalParameters  NCopyVariant=Disabled  FilterICVariant=InternalICsFilter  IntegratorICVariant=InternalICs  ExternalResetVariant=Disabled  TRSumVariant=Passthrough  SumFdbkVariant=Disabled  SumVariant=Sum_PID  TsampFilterVariant=InternalTs  TsampNgainVariant=Passthrough  TsampIntegralVariant=Passthrough  ExternalSaturationOutDataTypeStr=Inherit: Same as second input  aMode=0
  cfblk4 : DiscreteStateSpace
  cfblk5 : Product  Inputs=*
  cfblk6 : DotProduct  OutDataTypeStr=Inherit: Inherit via internal rule
  cfblk7 : Math  Operator=square
  cfblk8 : Product  Inputs=**
  cfblk9 : Constant  Value=[954416798.616567]  SampleTime=1
  cfblk2 : Outport
  cfblk13 : Outport  Port=2
  wires:
  cfblk9/1 -> cfblk2/1
  cfblk6/1 -> cfblk13/1
  cfblk4/1 -> cfblk5/1
  cfblk8/1 -> cfblk4/1
  cfblk3/1 -> cfblk8/1
  cfblk1/1 -> cfblk6/1
  cfblk12/1 -> cfblk8/2
  cfblk11/1 -> cfblk6/2
  cfblk10/1 -> cfblk7/1
  cfblk5/1 -> cfblk14/1
  cfblk14/1 -> cfblk3/1

== system sampleModel106/cfblk74/cfblk12/cfblk6/cfblk16 ==
  cfblk1 : Inport
  cfblk8 : Inport  Port=2
  cfblk9 : Inport  Port=3
  Action Port : ActionPort  ActionPortLabel=if(u1 >= 0)
  cfblk3 : DiscreteStateSpace  SampleTime=-1
  cfblk4 : DiscreteTransferFcn
  cfblk5 : Reshape
  cfblk6 : Sum  Inputs=+-
  cfblk7 : Rounding
  cfblk2 : Outport
  cfblk10 : Outport  Port=2
  wires:
  cfblk3/1 -> cfblk10/1
  cfblk1/1 -> cfblk6/1
  cfblk5/1 -> cfblk3/1
  cfblk8/1 -> cfblk4/1
  cfblk4/1 -> cfblk7/1
  cfblk9/1 -> cfblk6/2
  cfblk7/1 -> cfblk5/1
  cfblk6/1 -> cfblk2/1

== system sampleModel106/cfblk74/cfblk12/cfblk6/cfblk17 ==
  cfblk1 : Inport
  cfblk15 : Inport  Port=2
  cfblk16 : Inport  Port=3
  cfblk17 : Inport  Port=4
  Action Port : ActionPort  ActionPortLabel=else
  cfblk10 : Product  Inputs=**
  cfblk11 : Gain  Gain=[693236438.099026]
  cfblk12 : UnaryMinus
  cfblk13 : Constant  Value=[821940346.287199]  SampleTime=1
  cfblk14 : Constant  Value=[-263125850.057077]  SampleTime=1
  cfblk3 : simulink/Discrete/Transfer Fcn Lead or Lag  PoleZ=0.95  ZeroZ=0.75  ICPrevOutput=0.0  ICPrevInput=0.0  DoSatur=off
      settings: SourceProductBaseCode=SL
  cfblk4 : simulink/Discrete/Tapped Delay  vinit=0.0  samptime=-1  NumDelays=1  DelayOrder=Oldest  includeCurrent=off
  cfblk5 : Delay
  cfblk6 : Gain  Gain=[933869757.031214]
  cfblk7 : ComplexToRealImag
  cfblk8 : Rounding
  cfblk9 : Math  Operator=hypot
  cfblk2 : Outport
  wires:
  cfblk11/1 -> cfblk8/1
  cfblk7/1 -> cfblk6/1
  cfblk14/1 -> cfblk7/1
  cfblk5/1 -> cfblk10/1
  cfblk8/1 -> cfblk9/1
  cfblk13/1 -> cfblk11/1
  cfblk6/1 -> cfblk4/1
  cfblk4/1 -> cfblk2/1
  cfblk7/2 -> cfblk5/1
  cfblk15/1 -> cfblk9/2
  cfblk1/1 -> cfblk10/2
  cfblk16/1 -> cfblk3/1
  cfblk10/1 -> cfblk12/1

== system sampleModel106/cfblk74/cfblk12/cfblk7/cfblk7 ==
  cfblk1 : Inport
  cfblk13 : Inport  Port=2
  cfblk14 : Inport  Port=3
  cfblk10 : Product  Inputs=**
  cfblk11 : Constant  Value=[650292641.232246]  SampleTime=1
  cfblk12 : Constant  Value=[-103860920.706199]  SampleTime=1
  cfblk16 : Delay  SampleTime=1
  cfblk3 : DiscreteIntegrator  ICPrevOutput=DiscIntNeverNeededParam  ICPrevScaledInput=DiscIntNeverNeededParam
  cfblk4 : slpidlib/PID Controller  Controller=PID  Form=Parallel  TimeDomain=Discrete-time  UseExternalTs=off  SampleTime=1  IntegratorMethod=Forward Euler  FilterMethod=Forward Euler  ControllerParametersSource=internal  P=1  I=1  UseKiTs=off  D=0  N=100  UseFilter=on  TunerSelectOption=Transfer Function Based (PID Tuner App)  InitialConditionSource=internal  InitialConditionForIntegrator=0  InitialConditionForFilter=0  DifferentiatorICPrevScaledInput=0  ExternalReset=none  TrackingMode=off  Kt=1  LimitOutput=off  SatLimitsSource=internal  UpperSaturationLimit=inf  LowerSaturationLimit=-inf  LinearizeAsGain=off  AntiWindupMode=none  Kb=1  POutMin=[]  POutMax=[]  IOutMin=[]  IOutMax=[]  DOutMin=[]  DOutMax=[]  NOutMin=[]  NOutMax=[]  SumOutMin=[]  SumOutMax=[]  SaturationOutMin=[]  SaturationOutMax=[]  PParamMin=[]  PParamMax=[]  IParamMin=[]  IParamMax=[]  DParamMin=[]  DParamMax=[]  NParamMin=[]  NParamMax=[]  KbParamMin=[]  KbParamMax=[]  KtParamMin=[]  KtParamMax=[]  KbOutMin=[]  KbOutMax=[]  KtOutMin=[]  KtOutMax=[]  IntegratorOutMin=[]  IntegratorOutMax=[]  FilterOutMin=[]  FilterOutMax=[]  SumI1OutMin=[]  SumI1OutMax=[]  SumI2OutMin=[]  SumI2OutMax=[]  SumI3OutMin=[]  SumI3OutMax=[]  SumI4OutMin=[]  SumI4OutMax=[]  SumDOutMin=[]  SumDOutMax=[]  DifferentiatorOutMin=[]  DifferentiatorOutMax=[]  FilterDiffOutCoefMin=[]  FilterDiffOutCoefMax=[]  ReciprocalOutMin=[]  ReciprocalOutMax=[]  SumDenOutMin=[]  SumDenOutMax=[]  SumNumOutMin=[]  SumNumOutMax=[]  DivideOutMin=[]  DivideOutMax=[]  UdiffTsProdOutMin=[]  UdiffTsProdOutMax=[]  NTsProdOutMin=[]  NTsProdOutMax=[]  UintegralTsProdOutMin=[]  UintegralTsProdOutMax=[]  UngainTsProdOutMin=[]  UngainTsProdOutMax=[]  IntegratorContinuousStateAttributes=''  IntegratorStateMustResolveToSignalObject=off  IntegratorRTWStateStorageClass=Auto  FilterContinuousStateAttributes=''  FilterStateMustResolveToSignalObject=off  FilterRTWStateStorageClass=Auto  ParallelPVariant=InternalParameters  IdealPVariant=Disabled  IVariant=InternalParameters  DVariant=InternalParameters  IntegratorVariant=Discrete  SatVariant=Disabled  AWVariant=Passthrough  PCopyVariant=Disabled  TRVariant=Disabled  FdbkBlocksVariant=Forward  IdealPFdbkVariant=Disabled  SatFdbkVariant=Disabled  DerivativeFilterVariant=ForwardEulerFilter  NVariant=InternalParameters  NCopyVariant=Disabled  FilterICVariant=InternalICsFilter  IntegratorICVariant=InternalICs  ExternalResetVariant=Disabled  TRSumVariant=Passthrough  SumFdbkVariant=Disabled  SumVariant=Sum_PID  TsampFilterVariant=InternalTs  TsampNgainVariant=Passthrough  TsampIntegralVariant=Passthrough  ExternalSaturationOutDataTypeStr=Inherit: Same as second input  aMode=0
  cfblk5 : DiscreteFilter  SampleTime=1
  cfblk6 : Abs  SaturateOnIntegerOverflow=off
  cfblk7 : Trigonometry
  cfblk8 : Sum
  cfblk9 : DotProduct  OutDataTypeStr=Inherit: Inherit via internal rule
  cfblk2 : Outport
  cfblk15 : Outport  Port=2
  wires:
  cfblk5/1 -> cfblk9/1
  cfblk7/1 -> cfblk3/1
  cfblk13/1 -> cfblk4/1
  cfblk12/1 -> cfblk8/1
  cfblk6/1 -> cfblk15/1
  cfblk4/1 -> cfblk7/1
  cfblk1/1 -> cfblk8/2
  cfblk11/1 -> cfblk9/2
  cfblk9/1 -> cfblk10/1
  cfblk3/1 -> cfblk6/1
  cfblk14/1 -> cfblk10/2
  cfblk8/1 -> cfblk2/1
  cfblk10/1 -> cfblk16/1
  cfblk16/1 -> cfblk5/1

== system sampleModel106/cfblk74/cfblk12/cfblk8/cfblk8 ==
  cfblk1 : Inport
  cfblk3 : Product  Inputs=**
  cfblk4 : simulink/Math Operations/MinMax Running Resettable  Function=min  vinit=0.0
  cfblk5 : Trigonometry
  cfblk8 : Delay  SampleTime=1
  cfblk9 : Delay  SampleTime=1
  cfblk2 : Outport
  cfblk6 : Outport  Port=2
  cfblk7 : Outport  Port=3
  wires:
  cfblk1/1 -> cfblk5/1
  cfblk3/1 -> cfblk7/1, cfblk4/1, cfblk2/1, cfblk4/2
  cfblk5/1 -> cfblk6/1
  cfblk4/1 -> cfblk8/1, cfblk9/1
  cfblk8/1 -> cfblk3/1
  cfblk9/1 -> cfblk3/2

== system sampleModel106/cfblk74/cfblk13/cfblk11/cfblk10 ==
  cfblk1 : Inport
  cfblk9 : Inport  Port=2
  cfblk10 : Inport  Port=3
  cfblk3 : simulink/Discrete/Transfer Fcn Real Zero  ZeroZ=0.75  ICPrevInput=0.0  DoSatur=off
      settings: SourceProductBaseCode=SL
  cfblk4 : simulink/Discrete/Transfer Fcn Lead or Lag  PoleZ=0.95  ZeroZ=0.75  ICPrevOutput=0.0  ICPrevInput=0.0  DoSatur=off
      settings: SourceProductBaseCode=SL
  cfblk5 : DiscreteTransferFcn  SampleTime=1
  cfblk6 : Math  Operator=hypot
  cfblk7 : MinMax  Inputs=3
  cfblk8 : Sqrt  Operator=rSqrt  AlgorithmType=Newton-Raphson
  cfblk2 : Outport
  cfblk11 : Outport  Port=2
  cfblk12 : Outport  Port=3
  cfblk13 : Outport  Port=4
  cfblk14 : Outport  Port=5
  wires:
  cfblk3/1 -> cfblk8/1, cfblk7/3
  cfblk1/1 -> cfblk5/1
  cfblk5/1 -> cfblk4/1
  cfblk4/1 -> cfblk6/1, cfblk2/1
  cfblk6/1 -> cfblk3/1, cfblk7/2
  cfblk10/1 -> cfblk7/1
  cfblk7/1 -> cfblk13/1, cfblk14/1
  cfblk8/1 -> cfblk11/1
  cfblk9/1 -> cfblk12/1, cfblk6/2

== system sampleModel106/cfblk74/cfblk13/cfblk11/cfblk14 ==
  cfblk1 : Inport
  cfblk13 : Inport  Port=2
  cfblk14 : Inport  Port=3
  Action Port : ActionPort  ActionPortLabel=if(u1 >= 0)
  cfblk10 : Product
  cfblk11 : DotProduct  OutDataTypeStr=Inherit: Inherit via internal rule
  cfblk12 : Constant  Value=[701139018.675026]  SampleTime=1
  cfblk18 : Delay
  cfblk3 : ComplexToMagnitudeAngle
  cfblk4 : Assignment  DiagnosticForDimensions=Warning  IndexOptions=Index vector (dialog)  Indices=1  OutputSizes=1
  cfblk5 : Trigonometry
  cfblk6 : Product  Inputs=*
  cfblk7 : Math  Operator=mod
  cfblk8 : Product
  cfblk9 : Assignment  DiagnosticForDimensions=Warning  IndexOptions=Index vector (dialog)  Indices=1  OutputSizes=1
  cfblk2 : Outport
  cfblk15 : Outport  Port=2
  cfblk16 : Outport  Port=3
  cfblk17 : Outport  Port=4
  wires:
  cfblk4/1 -> cfblk11/1, cfblk11/2
  cfblk12/1 -> cfblk5/1, cfblk6/1
  cfblk7/1 -> cfblk10/1
  cfblk1/1 -> cfblk7/1
  cfblk14/1 -> cfblk8/1
  cfblk9/1 -> cfblk7/2
  cfblk10/1 -> cfblk15/1, cfblk3/1
  cfblk8/1 -> cfblk16/1, cfblk10/2
  cfblk6/1 -> cfblk2/1, cfblk9/2
  cfblk5/1 -> cfblk9/1
  cfblk3/1 -> cfblk17/1
  cfblk13/1 -> cfblk8/2
  cfblk3/2 -> cfblk4/2
  cfblk11/1 -> cfblk18/1
  cfblk18/1 -> cfblk4/1

== system sampleModel106/cfblk74/cfblk13/cfblk11/cfblk15 ==
  cfblk1 : Inport
  cfblk7 : Inport  Port=2
  cfblk8 : Inport  Port=3
  cfblk9 : Inport  Port=4
  cfblk10 : Inport  Port=5
  cfblk11 : Inport  Port=6
  Action Port : ActionPort  ActionPortLabel=else
  cfblk3 : Delay  DelayLengthSource=Input port
      settings: InputPortMap=u0,p1
  cfblk4 : simulink/Discrete/Transfer Fcn Real Zero  ZeroZ=0.75  ICPrevInput=0.0  DoSatur=off
      settings: SourceProductBaseCode=SL
  cfblk5 : DiscreteTransferFcn
  cfblk6 : Sin  TimeSource=Use external signal  SampleTime=0
  cfblk2 : Outport
  wires:
  cfblk9/1 -> cfblk5/1
  cfblk5/1 -> cfblk4/1
  cfblk1/1 -> cfblk2/1
  cfblk7/1 -> cfblk6/1
  cfblk11/1 -> cfblk3/1
  cfblk4/1 -> cfblk3/2

== system sampleModel106/cfblk74/cfblk13/cfblk11/cfblk7 ==
  cfblk1 : Inport
  cfblk11 : Inport  Port=2
  cfblk12 : Inport  Port=3
  cfblk13 : Inport  Port=4
  cfblk14 : Inport  Port=5
  cfblk15 : Inport  Port=6
  cfblk10 : Constant  Value=[-272827552.181540]  SampleTime=1
  cfblk3 : simulink/Discrete/Transfer Fcn First Order  PoleZ=0.95  ICPrevOutput=0.0  DoSatur=off
  cfblk4 : DotProduct  OutDataTypeStr=Inherit: Inherit via internal rule
  cfblk5 : Sqrt  Operator=rSqrt  AlgorithmType=Newton-Raphson
  cfblk6 : PermuteDimensions
  cfblk7 : Product  Inputs=**
  cfblk8 : Sin  TimeSource=Use external signal  SampleTime=0
  cfblk9 : Constant  Value=[412907284.954251]  SampleTime=1
  cfblk2 : Outport
  cfblk16 : Outport  Port=2
  wires:
  cfblk5/1 -> cfblk2/1
  cfblk12/1 -> cfblk6/1
  cfblk8/1 -> cfblk3/1
  cfblk14/1 -> cfblk16/1
  cfblk10/1 -> cfblk8/1
  cfblk3/1 -> cfblk5/1
  cfblk6/1 -> cfblk4/1
  cfblk11/1 -> cfblk4/2
  cfblk9/1 -> cfblk7/1
  cfblk4/1 -> cfblk7/2

== system sampleModel106/cfblk74/cfblk13/cfblk11/cfblk8 ==
  cfblk1 : Inport
  cfblk13 : Inport  Port=2
  cfblk14 : Inport  Port=3
  cfblk10 : simulink/Math Operations/MinMax Running Resettable  Function=min  vinit=0.0
  cfblk11 : Constant  Value=[-892290875.340503]  SampleTime=1
  cfblk12 : Constant  Value=[468769461.166075]  SampleTime=1
  cfblk3 : simulink/Discrete/Transfer Fcn Real Zero  ZeroZ=0.75  ICPrevInput=0.0  DoSatur=off
      settings: SourceProductBaseCode=SL
  cfblk4 : simulink/Discrete/Transfer Fcn Lead or Lag  PoleZ=0.95  ZeroZ=0.75  ICPrevOutput=0.0  ICPrevInput=0.0  DoSatur=off
      settings: SourceProductBaseCode=SL
  cfblk5 : simulink/Math Operations/MinMax Running Resettable  Function=min  vinit=0.0
  cfblk6 : Product
  cfblk7 : UnaryMinus
  cfblk8 : simulink/Math Operations/MinMax Running Resettable  Function=min  vinit=0.0
  cfblk9 : PermuteDimensions
  cfblk2 : Outport
  cfblk15 : Outport  Port=2
  wires:
  cfblk8/1 -> cfblk3/1
  cfblk4/1 -> cfblk7/1
  cfblk13/1 -> cfblk6/1
  cfblk11/1 -> cfblk4/1, cfblk8/2
  cfblk14/1 -> cfblk10/1
  cfblk3/1 -> cfblk9/1
  cfblk1/1 -> cfblk8/1
  cfblk6/1 -> cfblk10/2
  cfblk7/1 -> cfblk6/2
  cfblk12/1 -> cfblk2/1
  cfblk10/1 -> cfblk5/1
  cfblk9/1 -> cfblk5/2
  cfblk5/1 -> cfblk15/1
